simulink model "Aero_Workspace"  (R2021a)
settings: Solver=ode1be  StartTime=0.0  StopTime=inf  FixedStep=0.001  RelTol=1e-3  EnableMultiTasking=on
PreLoadFcn:
  | Aero_Workspace_Setup
model workspace (MAT data in the model file):
  Dg = 0.0071
  Dt = 0.158
  Jp = 0.022
  Mb = 1.3
  g = 9.81
values from neighbouring files (symbols this model uses):
  Kpp = 0.6*0.0154    (= 0.00924)    [Aero_Workspace_Parameters.m]
  Kpy = 2*0.00329    (= 0.00658)    [Aero_Workspace_Parameters.m]
  Kyp = -2.5*0.00167    (= -0.004175)    [Aero_Workspace_Parameters.m]
  Kyy = 0.0129    [Aero_Workspace_Parameters.m]
  Pitch_deg_range = 62    [Aero_Workspace_Setup.m]
undefined symbols (not defined in the file or in its folder): _AICAD8418WBRMZ_Default_sldprt, _AICBCR421UW67_Default_sldprt, _C0402100n25V_Default_sldprt, _C040210n25V_Default_sldprt, _C040212p50VC0G_Default_sldprt, _C06031u35V_Default_sldprt, _C06032u216V_Default_sldprt, _C100U50VEEEFC1H101P_Default_sldprt, _C12064u750V_01_sldprt, _C121010U50V_Default_sldprt, _COMMCYUSB2014BZXC_Default_sldprt, _COMMON_01_sldprt, _COMMON_Default_sldprt, _CONNFUSBBSMT_01_sldprt, _CONNMDF3A12P2DSA_Default_sldprt, _CONNMDF3A4P2DSA_Default_sldprt, _CONNMDF3A6P2DS_Default_sldprt, _CONNMDF3A9P2DS_Default_sldprt, _CONNMODULAR8P8CTOP_Default_sldprt, _CP6100U50VC0G_Default_sldprt, _CPLD5M80ZE64C5_Default_sldprt, _DB560C13F_01_sldprt, _Default_sldprt, _DSMBJ5361BTP_Default_sldprt, _EEPROMAT24CM01_Default_sldprt, _FBBLM21PG221SN1D_01_sldprt, _FBMPZ2012S601A_01_sldprt, _LED3mmRedGreenRA_Default_sldprt, _LEDLTRBGFSFRedGreenBlue_Default_sldprt, _LOGICNCP361SNT1G_Default_sldprt, _LOGICNOTSN74LVC3G14DCU_Default_sldprt, _OPL6206QTR_Default_sldprt, _OSC40000MHZ_Default_sldprt, _R0402100K_Default_sldprt, _R040210K0_Default_sldprt, _R04021K00_Default_sldprt, _R0402200R_Default_sldprt, _R040222R0_Default_sldprt, _R04026K04_Default_sldprt, _R0402DNP_Default_sldprt, _RA40R0_Default_sldprt, _RA41K005, _TP16258543_01_sldprt, _TVSUNI28V_Default_sldprt, _TVSUNI53V_Default_sldprt, _VREGAP733333SAG7_Default_sldprt, _VREGLTM8022EVPBF_Default_sldprt, _VREGPAM3112DAB120_Default_sldprt, _VREGTPS79318DBVR_01_sldprt, _XTAL192MHZNX2520SA_Default_sldprt, BGA121, CAP, CEEEFC1H101P, CONNFUSBBSMT, CONNMDF3A12P2DSA, CONNMDF3A4P2DSA, CONNMDF3A6P2DS, CONNMDF3A9P2DS, CONNModular8P8C, DDO214AA ... (+30)
libraries: sm_lib x1565, fl_lib x43, nesl_utility x22, quarc_library x12, simulink x2, ee_lib x2
(part 6 of 23)

== system Aero_Workspace/Virtual Aero/Simscape Multibody/Back Rotor - Motor 1/x06_Aero_Dynamic_Model_Fan_0_1_RIGID/C006_364_1_RIGID/C006_364_92_1_RIGID ==
  ReferenceFrame : sm_lib/Frames and Transforms/Reference Frame
  Solid : sm_lib/Body Elements/File Solid  ExtGeomFileName=C006-364-92_01_sldprt.STEP  UnitType=FromFile  ExtGeomFileUnits=m  StepReaderType=HEX  ExportConvexHullGeometry=off  InertiaType=Custom  Mass=smiData.Solid(166).mass  MassUnits=kg  CenterOfMass=smiData.Solid(166).CoM  CenterOfMassUnits=in  MomentsOfInertia=smiData.Solid(166).MoI  MomentsOfInertiaUnits=kg*in^2  ProductsOfInertia=smiData.Solid(166).PoI  ProductsOfInertiaUnits=kg*in^2  BasedOnType=Density  Density=1000  DensityUnits=kg/(m^3)  DoExposeReferenceFrame=on  SerializedFrames=<Frames/>  GraphicType=FromGeometry  MarkerShape=Sphere  MarkerSize=10  GraphicVisPropType=SimpleVisualProperties  GraphicDiffuseColor=smiData.Solid(166).color  GraphicSpecularColor=[0.5 0.5 0.5 1.0]  GraphicAmbientColor=[0.15 0.15 0.15 1.0]  GraphicEmissiveColor=[0.0 0.0 0.0 1.0]  GraphicShininess=75  GraphicOpacity=smiData.Solid(166).opacity
  F : PMIOPort  Side=Left
  connections:
  ReferenceFrame/RConn1 -- Solid/RConn1 -- F/RConn1

== system Aero_Workspace/Virtual Aero/Simscape Multibody/Back Rotor - Motor 1/x06_Aero_Dynamic_Model_Fan_0_1_RIGID/C006_364_1_RIGID/C006_364_93_1_RIGID ==
  ReferenceFrame : sm_lib/Frames and Transforms/Reference Frame
  Solid : sm_lib/Body Elements/File Solid  ExtGeomFileName=C006-364-93_01_sldprt.STEP  UnitType=FromFile  ExtGeomFileUnits=m  StepReaderType=HEX  ExportConvexHullGeometry=off  InertiaType=Custom  Mass=smiData.Solid(164).mass  MassUnits=kg  CenterOfMass=smiData.Solid(164).CoM  CenterOfMassUnits=in  MomentsOfInertia=smiData.Solid(164).MoI  MomentsOfInertiaUnits=kg*in^2  ProductsOfInertia=smiData.Solid(164).PoI  ProductsOfInertiaUnits=kg*in^2  BasedOnType=Density  Density=1000  DensityUnits=kg/(m^3)  DoExposeReferenceFrame=on  SerializedFrames=<Frames/>  GraphicType=FromGeometry  MarkerShape=Sphere  MarkerSize=10  GraphicVisPropType=SimpleVisualProperties  GraphicDiffuseColor=smiData.Solid(164).color  GraphicSpecularColor=[0.5 0.5 0.5 1.0]  GraphicAmbientColor=[0.15 0.15 0.15 1.0]  GraphicEmissiveColor=[0.0 0.0 0.0 1.0]  GraphicShininess=75  GraphicOpacity=smiData.Solid(164).opacity
  F : PMIOPort  Side=Left
  connections:
  Solid/RConn1 -- ReferenceFrame/RConn1 -- F/RConn1

== system Aero_Workspace/Virtual Aero/Simscape Multibody/Base/x01_Aero_Dynamic_Model_Base_1_RIGID/A002_675_2_RIGID/C006_121_1_RIGID ==
  C006_121_1_RIGID : Subsystem
  ReferenceFrame : sm_lib/Frames and Transforms/Reference Frame
  Transform : sm_lib/Frames and Transforms/Rigid Transform  TranslationMethod=Cartesian  TranslationStandardOffset=0  TranslationLengthUnit=in  TranslationStandardAxis=+Z  TranslationCartesianOffset=smiData.RigidTransform(357).translation  TranslationROffset=0  TranslationROffsetUnits=m  TranslationZOffset=0  TranslationZOffsetUnits=m  TranslationThetaOffset=0  TranslationThetaOffsetUnits=deg  RotationMethod=ArbitraryAxis  RotationAngleUnits=rad  RotationStandardAxis=+Z  RotationAngle=smiData.RigidTransform(357).angle  RotationArbitraryAxis=smiData.RigidTransform(357).axis  FollAlignAxisA=+X  BaseAlignAxisA=+Y  FollAlignAxisB=+Y  BaseAlignAxisB=+Z  RotationSequenceAxes=FollowerAxes  RotationSequence=XYX  RotationSequenceAngles=[0 0 0]  RotationSequenceAnglesUnits=deg  RotationMatrix=[1 0 0; 0 1 0; 0 0 1]
  Transform1 : sm_lib/Frames and Transforms/Rigid Transform  TranslationMethod=Cartesian  TranslationStandardOffset=0  TranslationLengthUnit=in  TranslationStandardAxis=+Z  TranslationCartesianOffset=smiData.RigidTransform(358).translation  TranslationROffset=0  TranslationROffsetUnits=m  TranslationZOffset=0  TranslationZOffsetUnits=m  TranslationThetaOffset=0  TranslationThetaOffsetUnits=deg  RotationMethod=ArbitraryAxis  RotationAngleUnits=rad  RotationStandardAxis=+Z  RotationAngle=smiData.RigidTransform(358).angle  RotationArbitraryAxis=smiData.RigidTransform(358).axis  FollAlignAxisA=+X  BaseAlignAxisA=+Y  FollAlignAxisB=+Y  BaseAlignAxisB=+Z  RotationSequenceAxes=FollowerAxes  RotationSequence=XYX  RotationSequenceAngles=[0 0 0]  RotationSequenceAnglesUnits=deg  RotationMatrix=[1 0 0; 0 1 0; 0 0 1]
  Transform2 : sm_lib/Frames and Transforms/Rigid Transform  TranslationMethod=Cartesian  TranslationStandardOffset=0  TranslationLengthUnit=in  TranslationStandardAxis=+Z  TranslationCartesianOffset=smiData.RigidTransform(359).translation  TranslationROffset=0  TranslationROffsetUnits=m  TranslationZOffset=0  TranslationZOffsetUnits=m  TranslationThetaOffset=0  TranslationThetaOffsetUnits=deg  RotationMethod=ArbitraryAxis  RotationAngleUnits=rad  RotationStandardAxis=+Z  RotationAngle=smiData.RigidTransform(359).angle  RotationArbitraryAxis=smiData.RigidTransform(359).axis  FollAlignAxisA=+X  BaseAlignAxisA=+Y  FollAlignAxisB=+Y  BaseAlignAxisB=+Z  RotationSequenceAxes=FollowerAxes  RotationSequence=XYX  RotationSequenceAngles=[0 0 0]  RotationSequenceAnglesUnits=deg  RotationMatrix=[1 0 0; 0 1 0; 0 0 1]
  Transform3 : sm_lib/Frames and Transforms/Rigid Transform  TranslationMethod=Cartesian  TranslationStandardOffset=0  TranslationLengthUnit=in  TranslationStandardAxis=+Z  TranslationCartesianOffset=smiData.RigidTransform(360).translation  TranslationROffset=0  TranslationROffsetUnits=m  TranslationZOffset=0  TranslationZOffsetUnits=m  TranslationThetaOffset=0  TranslationThetaOffsetUnits=deg  RotationMethod=ArbitraryAxis  RotationAngleUnits=rad  RotationStandardAxis=+Z  RotationAngle=smiData.RigidTransform(360).angle  RotationArbitraryAxis=smiData.RigidTransform(360).axis  FollAlignAxisA=+X  BaseAlignAxisA=+Y  FollAlignAxisB=+Y  BaseAlignAxisB=+Z  RotationSequenceAxes=FollowerAxes  RotationSequence=XYX  RotationSequenceAngles=[0 0 0]  RotationSequenceAnglesUnits=deg  RotationMatrix=[1 0 0; 0 1 0; 0 0 1]
  flush_stud_pmi_1_RIGID : Subsystem
  flush_stud_pmi_2_RIGID : Subsystem
  F : PMIOPort  Side=Right
  connections:
  C006_121_1_RIGID/LConn1 -- Transform/RConn1
  Transform1/RConn1 -- flush_stud_pmi_2_RIGID/LConn1
  Transform2/RConn1 -- flush_stud_pmi_1_RIGID/LConn1
  Transform/LConn1 -- ReferenceFrame/RConn1 -- Transform1/LConn1 -- Transform2/LConn1 -- Transform3/RConn1
  Transform3/LConn1 -- F/RConn1

== system Aero_Workspace/Virtual Aero/Simscape Multibody/Base/x01_Aero_Dynamic_Model_Base_1_RIGID/A002_675_2_RIGID/C006_126_1_RIGID ==
  C006_126_1_RIGID : Subsystem
  ReferenceFrame : sm_lib/Frames and Transforms/Reference Frame
  Transform : sm_lib/Frames and Transforms/Rigid Transform  TranslationMethod=Cartesian  TranslationStandardOffset=0  TranslationLengthUnit=in  TranslationStandardAxis=+Z  TranslationCartesianOffset=smiData.RigidTransform(351).translation  TranslationROffset=0  TranslationROffsetUnits=m  TranslationZOffset=0  TranslationZOffsetUnits=m  TranslationThetaOffset=0  TranslationThetaOffsetUnits=deg  RotationMethod=ArbitraryAxis  RotationAngleUnits=rad  RotationStandardAxis=+Z  RotationAngle=smiData.RigidTransform(351).angle  RotationArbitraryAxis=smiData.RigidTransform(351).axis  FollAlignAxisA=+X  BaseAlignAxisA=+Y  FollAlignAxisB=+Y  BaseAlignAxisB=+Z  RotationSequenceAxes=FollowerAxes  RotationSequence=XYX  RotationSequenceAngles=[0 0 0]  RotationSequenceAnglesUnits=deg  RotationMatrix=[1 0 0; 0 1 0; 0 0 1]
  Transform1 : sm_lib/Frames and Transforms/Rigid Transform  TranslationMethod=Cartesian  TranslationStandardOffset=0  TranslationLengthUnit=in  TranslationStandardAxis=+Z  TranslationCartesianOffset=smiData.RigidTransform(352).translation  TranslationROffset=0  TranslationROffsetUnits=m  TranslationZOffset=0  TranslationZOffsetUnits=m  TranslationThetaOffset=0  TranslationThetaOffsetUnits=deg  RotationMethod=ArbitraryAxis  RotationAngleUnits=rad  RotationStandardAxis=+Z  RotationAngle=smiData.RigidTransform(352).angle  RotationArbitraryAxis=smiData.RigidTransform(352).axis  FollAlignAxisA=+X  BaseAlignAxisA=+Y  FollAlignAxisB=+Y  BaseAlignAxisB=+Z  RotationSequenceAxes=FollowerAxes  RotationSequence=XYX  RotationSequenceAngles=[0 0 0]  RotationSequenceAnglesUnits=deg  RotationMatrix=[1 0 0; 0 1 0; 0 0 1]
  Transform2 : sm_lib/Frames and Transforms/Rigid Transform  TranslationMethod=Cartesian  TranslationStandardOffset=0  TranslationLengthUnit=in  TranslationStandardAxis=+Z  TranslationCartesianOffset=smiData.RigidTransform(353).translation  TranslationROffset=0  TranslationROffsetUnits=m  TranslationZOffset=0  TranslationZOffsetUnits=m  TranslationThetaOffset=0  TranslationThetaOffsetUnits=deg  RotationMethod=ArbitraryAxis  RotationAngleUnits=rad  RotationStandardAxis=+Z  RotationAngle=smiData.RigidTransform(353).angle  RotationArbitraryAxis=smiData.RigidTransform(353).axis  FollAlignAxisA=+X  BaseAlignAxisA=+Y  FollAlignAxisB=+Y  BaseAlignAxisB=+Z  RotationSequenceAxes=FollowerAxes  RotationSequence=XYX  RotationSequenceAngles=[0 0 0]  RotationSequenceAnglesUnits=deg  RotationMatrix=[1 0 0; 0 1 0; 0 0 1]
  Transform3 : sm_lib/Frames and Transforms/Rigid Transform  TranslationMethod=Cartesian  TranslationStandardOffset=0  TranslationLengthUnit=in  TranslationStandardAxis=+Z  TranslationCartesianOffset=smiData.RigidTransform(354).translation  TranslationROffset=0  TranslationROffsetUnits=m  TranslationZOffset=0  TranslationZOffsetUnits=m  TranslationThetaOffset=0  TranslationThetaOffsetUnits=deg  RotationMethod=ArbitraryAxis  RotationAngleUnits=rad  RotationStandardAxis=+Z  RotationAngle=smiData.RigidTransform(354).angle  RotationArbitraryAxis=smiData.RigidTransform(354).axis  FollAlignAxisA=+X  BaseAlignAxisA=+Y  FollAlignAxisB=+Y  BaseAlignAxisB=+Z  RotationSequenceAxes=FollowerAxes  RotationSequence=XYX  RotationSequenceAngles=[0 0 0]  RotationSequenceAnglesUnits=deg  RotationMatrix=[1 0 0; 0 1 0; 0 0 1]
  Transform4 : sm_lib/Frames and Transforms/Rigid Transform  TranslationMethod=Cartesian  TranslationStandardOffset=0  TranslationLengthUnit=in  TranslationStandardAxis=+Z  TranslationCartesianOffset=smiData.RigidTransform(355).translation  TranslationROffset=0  TranslationROffsetUnits=m  TranslationZOffset=0  TranslationZOffsetUnits=m  TranslationThetaOffset=0  TranslationThetaOffsetUnits=deg  RotationMethod=ArbitraryAxis  RotationAngleUnits=rad  RotationStandardAxis=+Z  RotationAngle=smiData.RigidTransform(355).angle  RotationArbitraryAxis=smiData.RigidTransform(355).axis  FollAlignAxisA=+X  BaseAlignAxisA=+Y  FollAlignAxisB=+Y  BaseAlignAxisB=+Z  RotationSequenceAxes=FollowerAxes  RotationSequence=XYX  RotationSequenceAngles=[0 0 0]  RotationSequenceAnglesUnits=deg  RotationMatrix=[1 0 0; 0 1 0; 0 0 1]
  Transform5 : sm_lib/Frames and Transforms/Rigid Transform  TranslationMethod=Cartesian  TranslationStandardOffset=0  TranslationLengthUnit=in  TranslationStandardAxis=+Z  TranslationCartesianOffset=smiData.RigidTransform(356).translation  TranslationROffset=0  TranslationROffsetUnits=m  TranslationZOffset=0  TranslationZOffsetUnits=m  TranslationThetaOffset=0  TranslationThetaOffsetUnits=deg  RotationMethod=ArbitraryAxis  RotationAngleUnits=rad  RotationStandardAxis=+Z  RotationAngle=smiData.RigidTransform(356).angle  RotationArbitraryAxis=smiData.RigidTransform(356).axis  FollAlignAxisA=+X  BaseAlignAxisA=+Y  FollAlignAxisB=+Y  BaseAlignAxisB=+Z  RotationSequenceAxes=FollowerAxes  RotationSequence=XYX  RotationSequenceAngles=[0 0 0]  RotationSequenceAnglesUnits=deg  RotationMatrix=[1 0 0; 0 1 0; 0 0 1]
  flush_stud_pmi_5_RIGID : Subsystem
  flush_stud_pmi_6_RIGID : Subsystem
  flush_stud_pmi_7_RIGID : Subsystem
  flush_stud_pmi_8_RIGID : Subsystem
  F : PMIOPort  Side=Right
  connections:
  Transform/RConn1 -- flush_stud_pmi_6_RIGID/LConn1
  Transform1/RConn1 -- flush_stud_pmi_7_RIGID/LConn1
  C006_126_1_RIGID/LConn1 -- Transform2/RConn1
  Transform3/RConn1 -- flush_stud_pmi_8_RIGID/LConn1
  Transform4/RConn1 -- flush_stud_pmi_5_RIGID/LConn1
  Transform/LConn1 -- ReferenceFrame/RConn1 -- Transform1/LConn1 -- Transform2/LConn1 -- Transform3/LConn1 -- Transform4/LConn1 -- Transform5/RConn1
  Transform5/LConn1 -- F/RConn1

== system Aero_Workspace/Virtual Aero/Simscape Multibody/Base/x01_Aero_Dynamic_Model_Base_1_RIGID/A002_675_2_RIGID/C006_127_1_RIGID ==
  ReferenceFrame : sm_lib/Frames and Transforms/Reference Frame
  Solid : sm_lib/Body Elements/File Solid  ExtGeomFileName=C006-127_01_sldprt.STEP  UnitType=FromFile  ExtGeomFileUnits=m  StepReaderType=HEX  ExportConvexHullGeometry=off  InertiaType=Custom  Mass=smiData.Solid(96).mass  MassUnits=kg  CenterOfMass=smiData.Solid(96).CoM  CenterOfMassUnits=in  MomentsOfInertia=smiData.Solid(96).MoI  MomentsOfInertiaUnits=kg*in^2  ProductsOfInertia=smiData.Solid(96).PoI  ProductsOfInertiaUnits=kg*in^2  BasedOnType=Density  Density=1000  DensityUnits=kg/(m^3)  DoExposeReferenceFrame=on  SerializedFrames=<Frames/>  GraphicType=FromGeometry  MarkerShape=Sphere  MarkerSize=10  GraphicVisPropType=SimpleVisualProperties  GraphicDiffuseColor=smiData.Solid(96).color  GraphicSpecularColor=[0.5 0.5 0.5 1.0]  GraphicAmbientColor=[0.15 0.15 0.15 1.0]  GraphicEmissiveColor=[0.0 0.0 0.0 1.0]  GraphicShininess=75  GraphicOpacity=smiData.Solid(96).opacity
  F : PMIOPort  Side=Left
  connections:
  Solid/RConn1 -- ReferenceFrame/RConn1 -- F/RConn1

== system Aero_Workspace/Virtual Aero/Simscape Multibody/Base/x01_Aero_Dynamic_Model_Base_1_RIGID/A002_675_2_RIGID/C006_128_1_RIGID ==
  ReferenceFrame : sm_lib/Frames and Transforms/Reference Frame
  Solid : sm_lib/Body Elements/File Solid  ExtGeomFileName=C006-128_01_sldprt.STEP  UnitType=FromFile  ExtGeomFileUnits=m  StepReaderType=HEX  ExportConvexHullGeometry=off  InertiaType=Custom  Mass=smiData.Solid(97).mass  MassUnits=kg  CenterOfMass=smiData.Solid(97).CoM  CenterOfMassUnits=in  MomentsOfInertia=smiData.Solid(97).MoI  MomentsOfInertiaUnits=kg*in^2  ProductsOfInertia=smiData.Solid(97).PoI  ProductsOfInertiaUnits=kg*in^2  BasedOnType=Density  Density=1000  DensityUnits=kg/(m^3)  DoExposeReferenceFrame=on  SerializedFrames=<Frames/>  GraphicType=FromGeometry  MarkerShape=Sphere  MarkerSize=10  GraphicVisPropType=SimpleVisualProperties  GraphicDiffuseColor=smiData.Solid(97).color  GraphicSpecularColor=[0.5 0.5 0.5 1.0]  GraphicAmbientColor=[0.15 0.15 0.15 1.0]  GraphicEmissiveColor=[0.0 0.0 0.0 1.0]  GraphicShininess=75  GraphicOpacity=smiData.Solid(97).opacity
  F : PMIOPort  Side=Left
  connections:
  Solid/RConn1 -- ReferenceFrame/RConn1 -- F/RConn1
